simulink model "quadrotor_emul_b"  (Simulink 7.9)
settings: Solver=ode45  StartTime=0.0  StopTime=inf  MaxStep=0.1  RelTol=1e-3
model workspace (MAT data in the model file):
  server = []
InitFcn:
  | % load parameters of the default quadrotor
  | disp('Quadrotor parameters loaded by InitFcn')
  | mdl_quadcopter
undefined symbols (not defined in the file or in its folder): quad
libraries: roblocks x3
settings Model: Creator=corkep  LastModifiedBy=fehu
settings OptimizationCC: OptimizeModelRefInitCode=on  LifeSpan=Inf
settings DebuggingCC: StrictBusMsg=Warning
settings HardwareCC: ProdBitPerInt=16  ProdBitPerPointer=8  ProdIntDivRoundTo=Zero  ProdEndianess=LittleEndian  ProdWordSize=8  ProdHWDeviceType=Atmel->AVR
settings RTWCC: SystemTargetFile=realtime.tlc  GenerateMakefile=off  TemplateMakefile=realtime.tmf  Description=Real-Time Toolbox  RTWVerbose=off  ProcessScript=realtime_make_rtw_hook
settings CodeAppCC: IgnoreCustomStorageClasses=off
settings STFCustomTargetCC: TargetLibSuffix=.a  CodeReplacementLibrary=ANSI_C  GenerateSampleERTMain=on  CombineOutputUpdateFcns=on  ERTCustomFileBanners=on  SupportContinuousTime=off  SupportNonInlinedSFcns=off  GRTInterface=off  SystemTargetFile=realtime.tlc
settings ERTTargetCC: CodeReplacementLibrary=ANSI_C  MultiwordLength=2048  GenerateSampleERTMain=on  ParMdlRefBuildCompliant=off  CompOptLevelCompliant=off  ConcurrentExecutionCompliant=off  ERTFirstTimeCompliant=off  ModelStepFunctionPrototypeControlCompliant=off  CPPClassGenCompliant=off  InlinedParameterPlacement=NonHierarchical  ERTCustomFileTemplate=realtime_file_process.tlc  ConvertIfToSwitch=off  SuppressUnreachableDefaultCases=off
settings SettingsController: Description=Run on Hardware Dialog  TargetExtensionPlatform=None

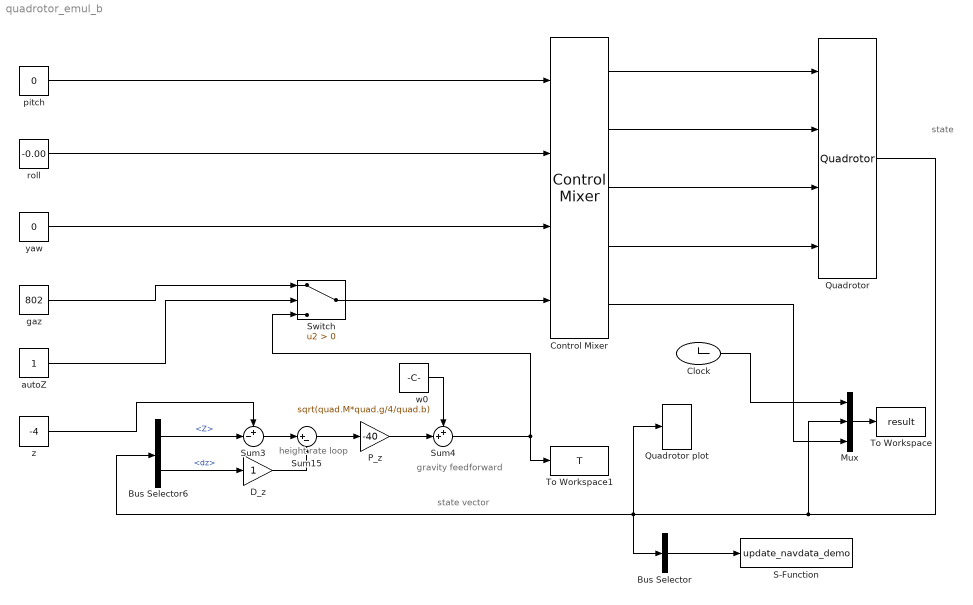
== system quadrotor_emul_b ==
  note: state vector
  note: gravity feedforward
  note: height rate
      | loop
  note: state
  Bus Selector : BusSelector  OutputSignals=dx,dy,dz,droll,dpitch,dyaw,Z  OutputAsBus=on
  Bus Selector6 : BusSelector  OutputSignals=Z,dz
  Clock : Clock
  Control Mixer : roblocks/Dynamics/Control Mixer
  D_z : Gain
  Mux : Mux  Inputs=3
  P_z : Gain  Gain=-40
  Quadrotor : roblocks/Dynamics/Quadrotor  quad=quad
  Quadrotor plot : roblocks/Robot Graphics/Quadrotor plot  RequirementInfo="{}  %GIDa_636c0778_5e43_4edb_8038_f3f250d9dd7b"  x=0
  S-Function : S-Function  FunctionName=update_navdata_demo  EnableBusSupport=off
  Sum15 : Sum  Inputs=|+-
  Sum3 : Sum  Inputs=+-|
  Sum4 : Sum  Inputs=++|
  Switch : Switch  Criteria=u2 > Threshold
  To Workspace : ToWorkspace  VariableName=result  SampleTime=-1
  To Workspace1 : ToWorkspace  VariableName=T  SampleTime=-1
  autoZ : Constant
  gaz : Constant  Value=802
  pitch : Constant  Value=0
  roll : Constant  Value=-0.00
  w0 : Constant  Value=sqrt(quad.M*quad.g/4/quad.b)  SampleTime=0
  yaw : Constant  Value=0
  z : Constant  Value=-4
  wires:
  Control Mixer/1 -> Quadrotor/1
  Control Mixer/4 -> Quadrotor/4
  w0/1 -> Sum4/1
  Sum15/1 -> P_z/1
  P_z/1 -> Sum4/2
  Quadrotor/1 -> Quadrotor plot/1, Bus Selector6/1, Bus Selector/1, Mux/2
  Bus Selector6/1 -> Sum3/2  "<Z>"
  z/1 -> Sum3/1
  Sum3/1 -> Sum15/1
  Bus Selector6/2 -> D_z/1  "<dz>"
  D_z/1 -> Sum15/2
  Sum4/1 -> To Workspace1/1, Switch/3
  Mux/1 -> To Workspace/1
  Clock/1 -> Mux/1
  Control Mixer/5 -> Mux/3
  yaw/1 -> Control Mixer/3
  Control Mixer/3 -> Quadrotor/3
  Control Mixer/2 -> Quadrotor/2
  roll/1 -> Control Mixer/2
  pitch/1 -> Control Mixer/1
  autoZ/1 -> Switch/2
  Switch/1 -> Control Mixer/4
  gaz/1 -> Switch/1
  Bus Selector/1 -> S-Function/1
